simulink model "incremental_rst_sim"  (R2023a)
settings: Solver=VariableStepAuto  StartTime=0.0  StopTime=3600  RelTol=1e-3
values from neighbouring files (symbols this model uses):
  ts = 5    [digital_control.m]
undefined symbols (not defined in the file or in its folder): A_hum, A_tot, Acv, Anet, Ar, As, Awi, bf, cp_b, cp_co, cpa, cpa_skin, cpm, cpw, eps_s, epsilon_w, Evap, h_m_hum, hacv, hf_g, hfg, hscv, IV, K_c, Kmat, m, maire, mco, mdot_a, ms, mw, P_atm, Qmet, r, R_hum, rho_a, rho_bl, rho_c, rho_w, s, Sa, sigma, thm, V_aire, Vb, Wex
settings Model: Creator=ACER  LastModifiedBy=ACER

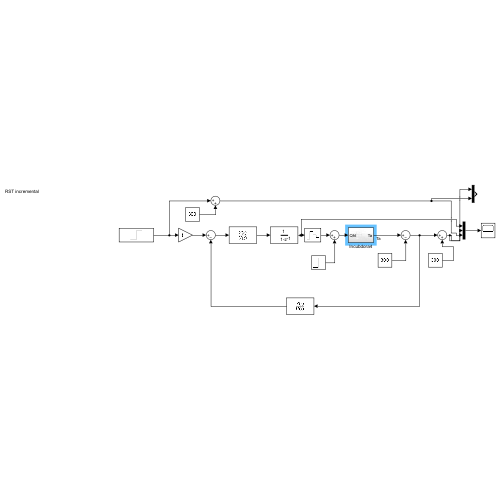
[thumbnail: Simulink's stored preview of the top-level diagram]
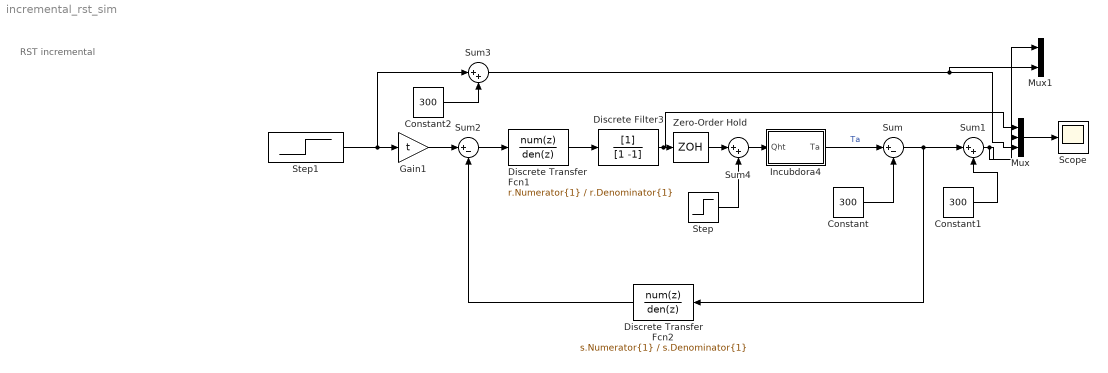
== system incremental_rst_sim ==
  note: RST incremental
  Constant : Constant  Value=300
  Constant1 : Constant  Value=300
  Constant2 : Constant  Value=300
  Discrete Transfer Fcn1 : DiscreteTransferFcn  Numerator=r.Numerator{1}  Denominator=r.Denominator{1}  SampleTime=ts
  Discrete Transfer Fcn2 : DiscreteTransferFcn  Numerator=s.Numerator{1}  Denominator=s.Denominator{1}  SampleTime=ts
  Discrete Filter3 : DiscreteFilter  Denominator=[1 -1]
  Gain1 : Gain  Gain=t
  Incubdora4 : Subsystem
  Mux : Mux  Inputs=3
  Mux1 : Mux  Inputs=2
  Scope : Scope
  Step : Step  Time=2000  After=0  SampleTime=0
  Step1 : Step  Time=0  After=10  SampleTime=0
  Sum : Sum  Inputs=|+-
  Sum1 : Sum  Inputs=|++
  Sum2 : Sum  Inputs=|+-
  Sum3 : Sum  Inputs=|++
  Sum4 : Sum  Inputs=|++
  Zero-Order Hold : ZeroOrderHold  SampleTime=-1
  wires:
  Step1/1 -> Sum3/1, Gain1/1
  Sum2/1 -> Discrete Transfer Fcn1/1
  Discrete Transfer Fcn2/1 -> Sum2/2
  Discrete Transfer Fcn1/1 -> Discrete Filter3/1
  Gain1/1 -> Sum2/1
  Discrete Filter3/1 -> Mux/1, Zero-Order Hold/1
  Sum1/1 -> Mux1/1, Mux/2
  Constant1/1 -> Sum1/2
  Constant2/1 -> Sum3/2
  Sum3/1 -> Mux1/2, Mux/3
  Mux/1 -> Scope/1
  Sum/1 -> Discrete Transfer Fcn2/1, Sum1/1
  Incubdora4/1(Ta) -> Sum/1  "Ta"
  Constant/1 -> Sum/2
  Zero-Order Hold/1 -> Sum4/1
  Sum4/1 -> Incubdora4/1(Qht)
  Step/1 -> Sum4/2

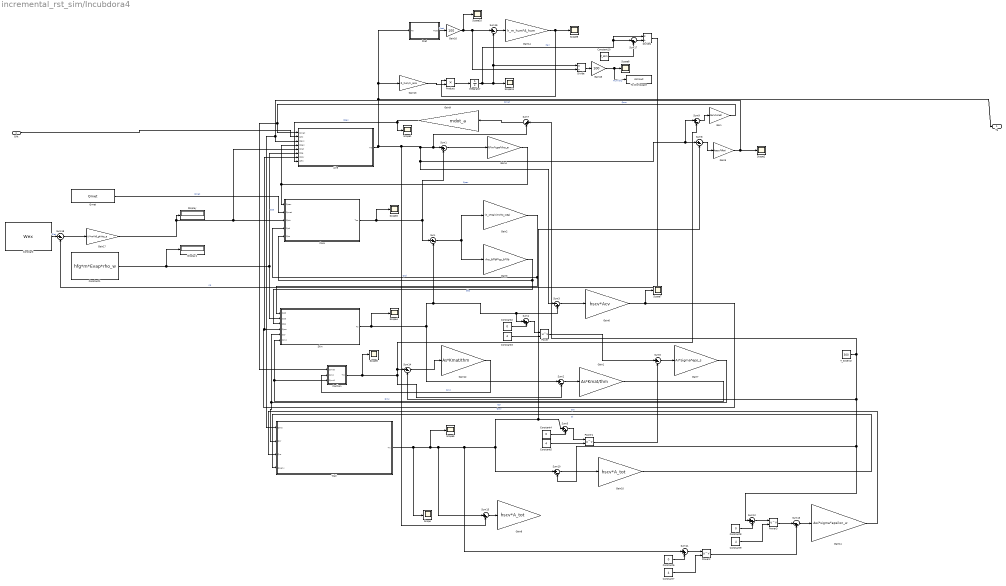
== system incremental_rst_sim/Incubdora4 ==
  Qht : Inport
  Aire : Subsystem
  Coclhon : Subsystem
  Constant : Constant  Value=Wex
  Constant1 : Constant  Value=hfg*m*Evap*rho_w
  Constant10 : Constant  Value=P_atm
  Constant{2,4,6,8} (4 alike) : Constant  Value=0
  Constant{3,5,7,9} (4 alike) : Constant  Value=4
  Core : Subsystem
  Display : Display
  Display1 : Display
  Divide : Product  Inputs=*/
  Divide1 : Product  Inputs=*/
  Gain : Gain  Gain=hacv*Anet
  Gain1 : Gain  Gain=As*Kmat/thm
  Gain10 : Gain  Gain=hscv*A_tot
  Gain11 : Gain  Gain=Awi*sigma*epsilon_w
  Gain12 : Gain  Gain=As*Kmat/thm
  Gain13 : Gain  Gain=R_hum/V_aire
  Gain14 : Gain  Gain=h_m_hum*A_hum
  Gain15 : Gain  Gain=100
  Gain16 : Gain  Gain=100
  Gain17 : Gain  Gain=IV*m*hf_g*rho_a
  Gain2 : Gain  Gain=(K_c*Sa)/(m/rho_c/Sa)
  Gain3 : Gain  Gain=rho_bl*bf*cp_b*Vb
  Gain4 : Gain  Gain=IV*m*cpa*rho_a
  Gain5 : Gain  Gain=hacv*Awi
  Gain6 : Gain  Gain=hscv*Acv
  Gain7 : Gain  Gain=Ar*sigma*eps_s
  Gain8 : Gain  Gain=hscv*A_tot
  Gain9 : Gain  Gain=mdot_a
  Integrator : Integrator
  Power{,1..3} (4 alike) : Math  Operator=pow
  Product : Product
  Psat : Subsystem
  Qmet : Constant  Value=Qmet
  Scope{,1..11} (12 alike) : Scope
  Skin : Subsystem
  Sum{,2,6..10,14..16,18} (11 alike) : Sum  Inputs=|+-
  Sum{1,3,13,17} (4 alike) : Sum  Inputs=|-+
  Sum{4..5,11..12} (4 alike) : Sum  Inputs=|++
  T_exterior : Constant  Value=300
  To Workspace : ToWorkspace  VariableName=simout  SaveFormat=Timeseries  SampleTime=-1
  Wall : Subsystem
  Ta : Outport
  wires:
  Gain/1 -> Aire/1(Qmat), Coclhon/1(Qmat)  "Qmat"
  Gain5/1 -> Scope2/1, Wall/1(Qacv), Aire/3(Qacv)  "Qacv"
  Power/1 -> Sum6/1
  Gain2/1 -> Skin/1(Qcd), Core/4(Qcd)  "Qcd"
  Sum1/1 -> Gain4/1
  Constant3/1 -> Power/2
  Aire/1(Ta) -> Ta/1, Psat/1(Ta), Gain13/1, Sum15/2, Sum9/1, Sum8/1, Sum3/1, Sum7/2, Sum1/1
  Qmet/1 -> Core/2(Qmet)  "Qmet"
  Power1/1 -> Sum6/2
  Sum4/1 -> Power/1
  Sum3/1 -> Gain6/1
  Sum14/1 -> Gain12/1
  Sum5/1 -> Power1/1
  Constant2/1 -> Sum4/2
  Gain7/1 -> Wall/2(Qsr), Skin/5(Qsr)  "Qsr"
  Gain4/1 -> Aire/4(Qsen), Core/1(Qsen)  "Qsen"
  Constant1/1 -> Display1/1, Skin/2(Qse), Aire/6(Qse)  "Qse"
  Sum/1 -> Gain3/1, Gain2/1
  Gain11/1 -> Wall/3(Qro)  "Qro"
  Sum13/1 -> Gain11/1
  Constant8/1 -> Sum12/2
  Gain1/1 -> Skin/6(Qmc), Coclhon/3(Qmc1)  "Qmc"
  Core/1(Tco) -> Scope3/1, Sum1/2, Sum/1
  Constant4/1 -> Sum5/2
  Wall/1(Tw) -> Scope/1, Sum10/1, Sum8/2, Sum5/1, Sum11/1, Sum15/1, Scope5/1
  Skin/1(Ts) -> Scope4/1, Sum4/1, Sum3/2, Sum/2, Sum2/1
  Constant5/1 -> Power1/2
  Constant6/1 -> Sum11/2
  Sum2/1 -> Gain1/1
  Gain6/1 -> Scope7/1, Aire/7(Qscv), Skin/4(Qscv)  "Qscv"
  Gain3/1 -> Skin/3(Qbc), Core/5(Qbc)  "Qbc"
  Sum8/1 -> Gain5/1
  Power2/1 -> Sum13/2
  T_exterior/1 -> Sum14/2, Sum10/2, Sum12/1, Sum7/1
  Sum12/1 -> Power3/1
  Constant7/1 -> Power2/2
  Constant9/1 -> Power3/2
  Sum6/1 -> Gain7/1
  Sum9/1 -> Gain/1
  Sum11/1 -> Power2/1
  Power3/1 -> Sum13/1
  Coclhon/1(Tm) -> Scope6/1, Sum2/2, Sum14/1, Sum9/2
  Qht/1 -> Aire/2(Qht)
  Gain12/1 -> Coclhon/2(Qmc)  "Qmc"
  Sum7/1 -> Gain9/1
  Gain9/1 -> Scope1/1, Aire/8(Qfm)  "Qsen"
  Sum15/1 -> Gain8/1
  Gain10/1 -> Wall/4(Qoenv)  "Qi"
  Sum10/1 -> Gain10/1
  Psat/1(Psat) -> Gain16/1  "Psat"
  Integrator/1 -> Divide1/1, Sum17/1, Scope11/1, Divide/1, Sum16/2  "Pair"
  Sum16/1 -> Gain14/1
  Gain13/1 -> Product/2
  Product/1 -> Integrator/1
  Gain14/1 -> Scope9/1, Product/1
  Divide/1 -> Gain15/1
  Gain15/1 -> To Workspace/1, Scope8/1  "Humidity"
  Gain16/1 -> Scope10/1, Divide/2, Sum16/1
  Constant10/1 -> Sum17/2
  Sum17/1 -> Divide1/2
  Divide1/1 -> Sum18/2  "wa"
  Constant/1 -> Sum18/1  "Qlat"
  Sum18/1 -> Gain17/1
  Gain17/1 -> Aire/5(Qlat), Core/3(Qlat), Display/1

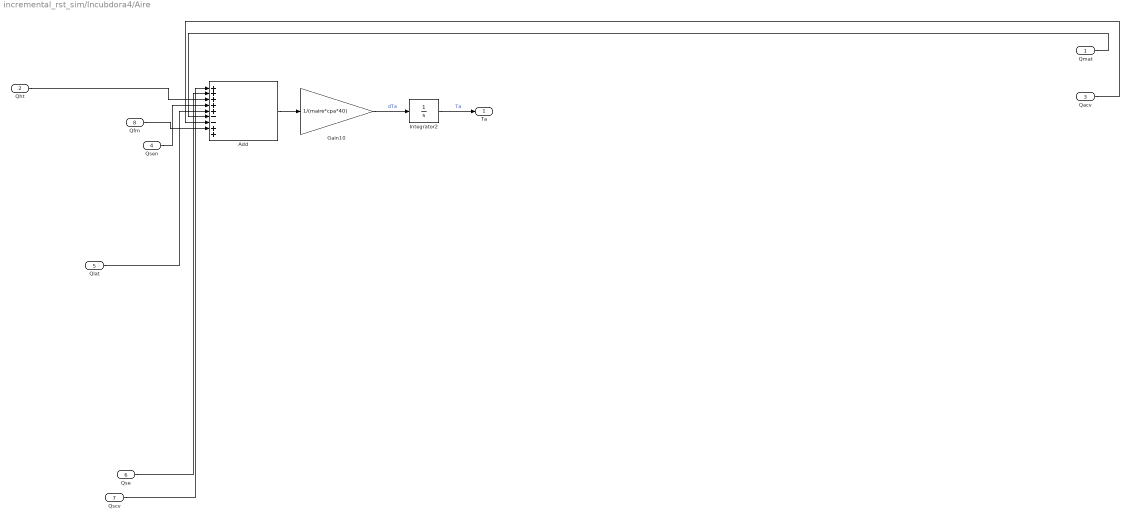
== system incremental_rst_sim/Incubdora4/Aire ==
  Qmat : Inport
  Qht : Inport  Port=2
  Qacv : Inport  Port=3
  Qsen : Inport  Port=4
  Qlat : Inport  Port=5
  Qse : Inport  Port=6
  Qscv : Inport  Port=7
  Qfm : Inport  Port=8
  Add : Sum  Inputs=+++++--++
  Gain10 : Gain  Gain=1/(maire*cpa*40)
  Integrator2 : Integrator  InitialCondition=300
  Ta : Outport
  wires:
  Qse/1 -> Add/2
  Qsen/1 -> Add/4
  Qlat/1 -> Add/5
  Add/1 -> Gain10/1
  Integrator2/1 -> Ta/1  "Ta"
  Gain10/1 -> Integrator2/1  "dTa"
  Qscv/1 -> Add/1
  Qacv/1 -> Add/7
  Qmat/1 -> Add/6
  Qht/1 -> Add/3
  Qfm/1 -> Add/8

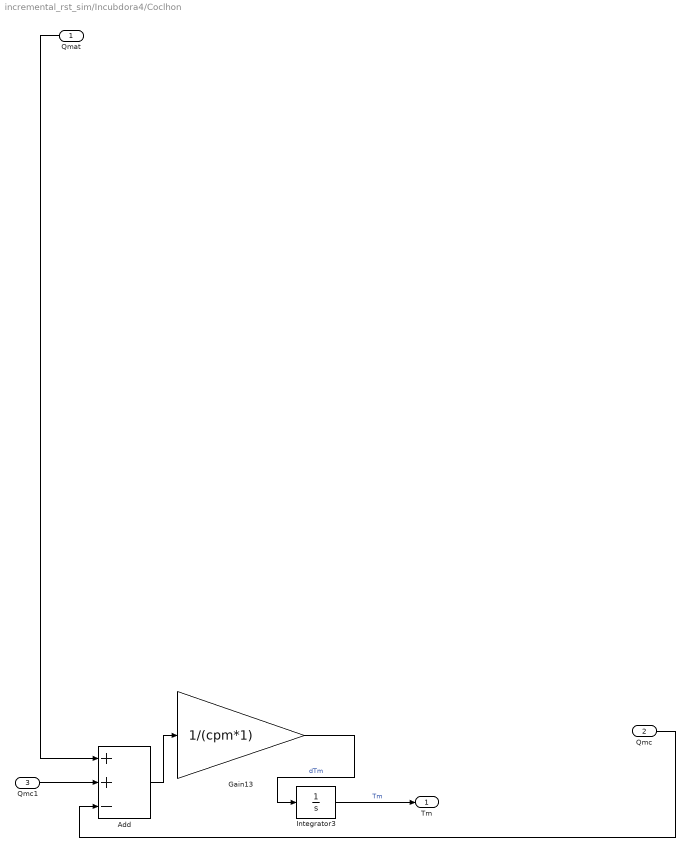
== system incremental_rst_sim/Incubdora4/Coclhon ==
  Qmat : Inport
  Qmc : Inport  Port=2
  Qmc1 : Inport  Port=3
  Add : Sum  Inputs=++-
  Gain13 : Gain  Gain=1/(cpm*1)
  Integrator3 : Integrator  InitialCondition=300
  Tm : Outport
  wires:
  Integrator3/1 -> Tm/1  "Tm"
  Add/1 -> Gain13/1
  Gain13/1 -> Integrator3/1  "dTm"
  Qmc/1 -> Add/3
  Qmat/1 -> Add/1
  Qmc1/1 -> Add/2

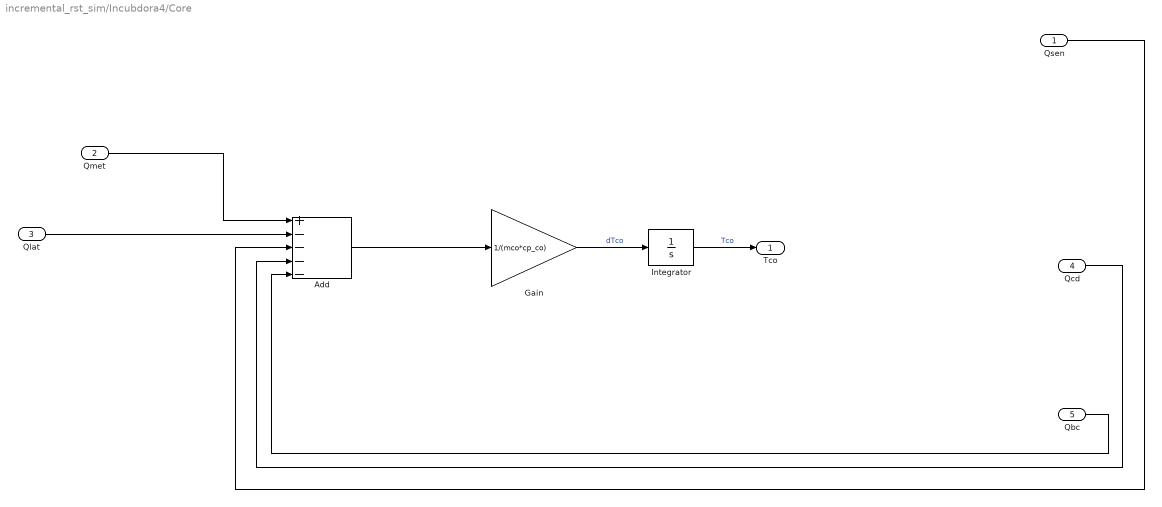
== system incremental_rst_sim/Incubdora4/Core ==
  Qsen : Inport
  Qmet : Inport  Port=2
  Qlat : Inport  Port=3
  Qcd : Inport  Port=4
  Qbc : Inport  Port=5
  Add : Sum  Inputs=+----
  Gain : Gain  Gain=1/(mco*cp_co)
  Integrator : Integrator  InitialCondition=308
  Tco : Outport
  wires:
  Qlat/1 -> Add/2
  Gain/1 -> Integrator/1  "dTco"
  Qbc/1 -> Add/5
  Qcd/1 -> Add/4
  Integrator/1 -> Tco/1  "Tco"
  Add/1 -> Gain/1
  Qmet/1 -> Add/1
  Qsen/1 -> Add/3

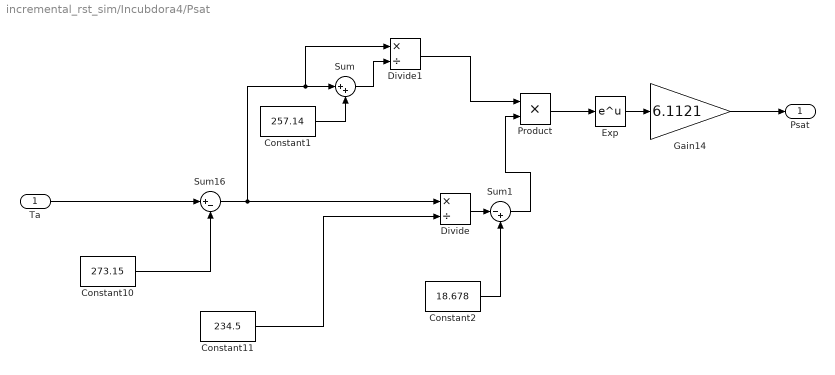
== system incremental_rst_sim/Incubdora4/Psat ==
  Ta : Inport
  Constant1 : Constant  Value=257.14
  Constant10 : Constant  Value=273.15
  Constant11 : Constant  Value=234.5
  Constant2 : Constant  Value=18.678
  Divide : Product  Inputs=*/
  Divide1 : Product  Inputs=*/
  Exp : Math
  Gain14 : Gain  Gain=6.1121
  Product : Product
  Sum : Sum  Inputs=|++
  Sum1 : Sum  Inputs=|-+
  Sum16 : Sum  Inputs=|+-
  Psat : Outport
  wires:
  Constant11/1 -> Divide/2
  Gain14/1 -> Psat/1
  Constant10/1 -> Sum16/2
  Ta/1 -> Sum16/1
  Sum16/1 -> Divide1/1, Sum/1, Divide/1
  Constant1/1 -> Sum/2
  Sum/1 -> Divide1/2
  Divide1/1 -> Product/1
  Constant2/1 -> Sum1/2
  Product/1 -> Exp/1
  Exp/1 -> Gain14/1
  Divide/1 -> Sum1/1
  Sum1/1 -> Product/2

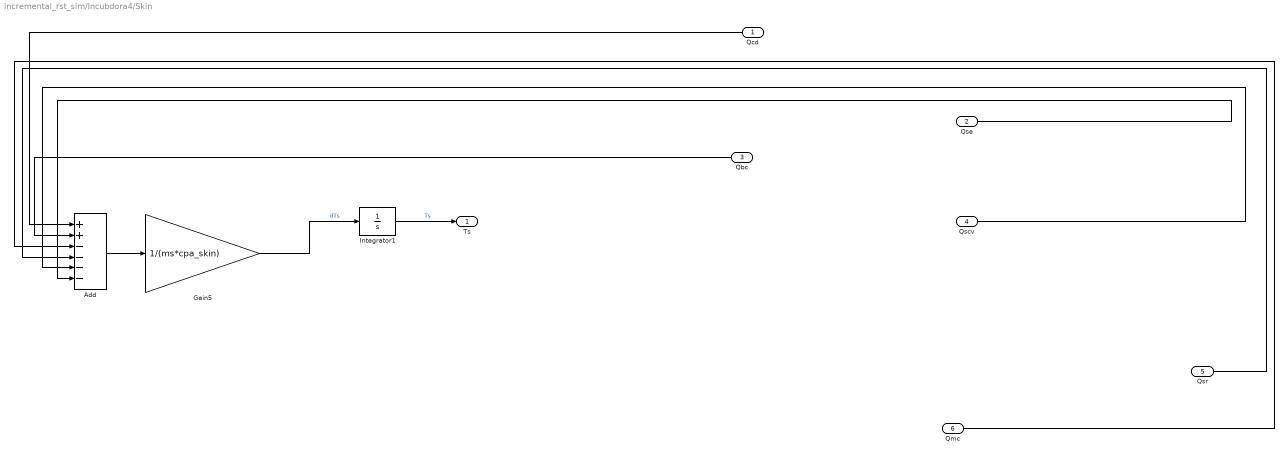
== system incremental_rst_sim/Incubdora4/Skin ==
  Qcd : Inport
  Qse : Inport  Port=2
  Qbc : Inport  Port=3
  Qscv : Inport  Port=4
  Qsr : Inport  Port=5
  Qmc : Inport  Port=6
  Add : Sum  Inputs=++----
  Gain5 : Gain  Gain=1/(ms*cpa_skin)
  Integrator1 : Integrator  InitialCondition=308
  Ts : Outport
  wires:
  Qbc/1 -> Add/2
  Qscv/1 -> Add/5
  Add/1 -> Gain5/1
  Gain5/1 -> Integrator1/1  "dTs"
  Qse/1 -> Add/6
  Qmc/1 -> Add/3
  Qsr/1 -> Add/4
  Integrator1/1 -> Ts/1  "Ts"
  Qcd/1 -> Add/1

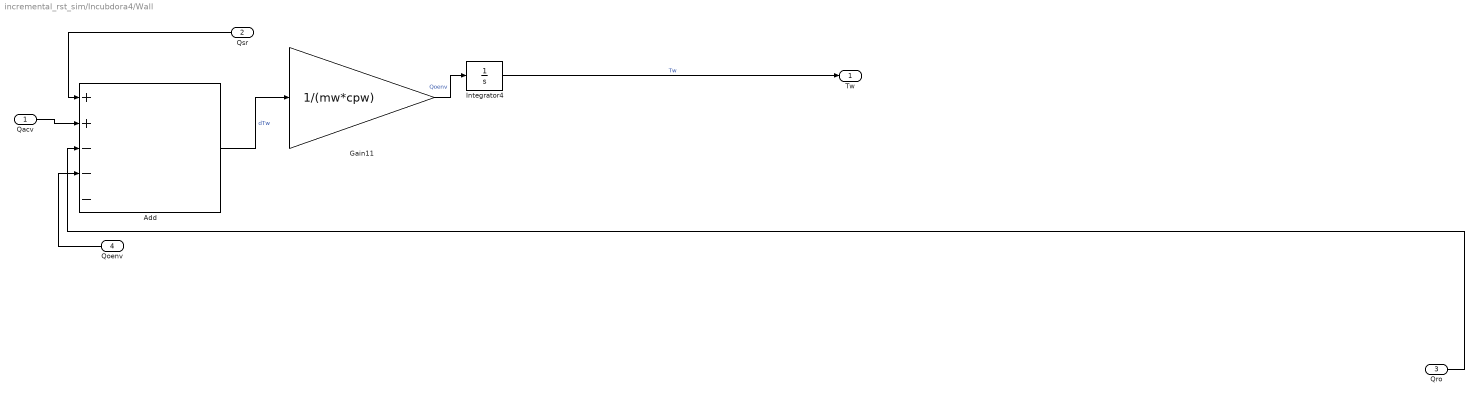
== system incremental_rst_sim/Incubdora4/Wall ==
  Qacv : Inport
  Qsr : Inport  Port=2
  Qro : Inport  Port=3
  Qoenv : Inport  Port=4
  Add : Sum  Inputs=++---
  Gain11 : Gain  Gain=1/(mw*cpw)
  Integrator4 : Integrator  InitialCondition=300
  Tw : Outport
  wires:
  Add/1 -> Gain11/1  "dTw"
  Qsr/1 -> Add/1
  Qacv/1 -> Add/2
  Gain11/1 -> Integrator4/1  "Qoenv"
  Qro/1 -> Add/3
  Integrator4/1 -> Tw/1  "Tw"
  Qoenv/1 -> Add/4
